simulink model "linear2DOF"  (R2025b)
settings: Solver=FixedStepAuto  StartTime=0.0  StopTime=1000  FixedStep=0.001  RelTol=1e-3
InitFcn:
  | % 定义车辆参数
  | m = 1370 + 89.9 + 65.2 + 22*4;       % 车辆质量 (kg)
  | Vx = 120/3.6;        % 纵向速度 (m/s)
  | Cf = -4.487763550086564e+04 * 2;    % 前轴总侧偏刚度 (N/rad)
  | Cr = Cf;   % 后轴总侧偏刚度 (N/rad)
  | lf = 1.11;       % 质心到前轴距离 (m)
  | lr = 2.866-lf;       % 质心到后轴距离 (m)
  | Iz = 2315.3 + 0.08 + 0.08 + 0.8*4;      % 绕z轴转动惯量 (kg·m²)
undefined symbols (not defined in the file): speed_from_matlab
libraries: Solver_SF x1
settings Model: Creator=23649  LastModifiedBy=23649

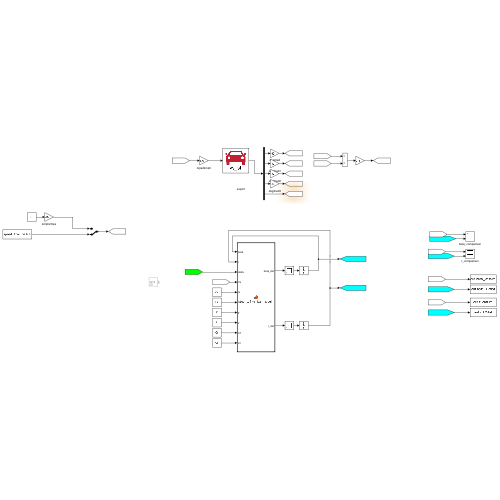
[thumbnail: Simulink's stored preview of the top-level diagram]
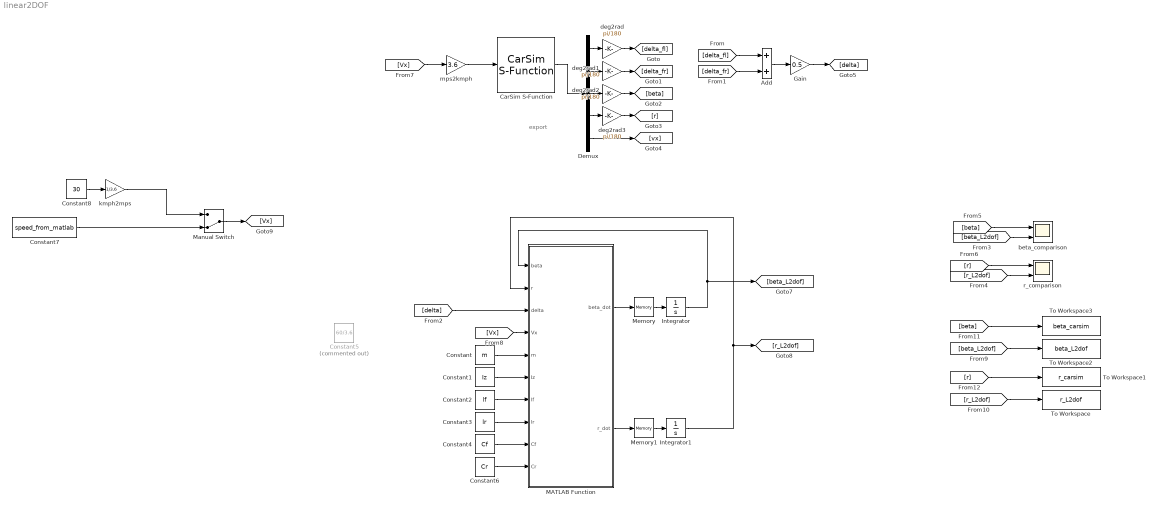
== system linear2DOF ==
  note: export
  Add : Sum
  CarSim S-Function : Solver_SF/CarSim S-Function  Priority=1  SIMFILE=simfile.sim  Run_RTs=off  vs_state_ind=Run  StopMode_ind=Vehicle Model
  Constant : Constant  Value=m
  Constant1 : Constant  Value=Iz
  Constant2 : Constant  Value=lf
  Constant3 : Constant  Value=lr
  Constant4 : Constant  Value=Cf
  Constant5 : Constant  Commented=on  Value=60/3.6
  Constant6 : Constant  Value=Cr
  Constant7 : Constant  Value=speed_from_matlab
  Constant8 : Constant  Value=30
  Demux : Demux  Outputs=5
  Gain : Gain  Gain=0.5
  Integrator : Integrator
  Integrator1 : Integrator
  MATLAB Function : MATLAB Function  TreatAsAtomicUnit=on
  Manual Switch : ManualSwitch  CurrentSetting=0
  Memory : Memory
  Memory1 : Memory
  To Workspace : ToWorkspace  VariableName=r_L2dof  SampleTime=-1
  To Workspace1 : ToWorkspace  VariableName=r_carsim  SampleTime=-1
  To Workspace2 : ToWorkspace  VariableName=beta_L2dof  SampleTime=-1
  To Workspace3 : ToWorkspace  VariableName=beta_carsim  SampleTime=-1
  beta_comparison : Scope  NumInputPorts=2
      settings: ActiveDisplayYMinimum=-1  ActiveDisplayYMaximum=1
  deg2rad{,1..3} (4 alike) : Gain  Gain=pi/180
  kmph2mps : Gain  Gain=1/3.6
  mps2kmph : Gain  Gain=3.6
  r_comparison : Scope  NumInputPorts=2
      settings: ActiveDisplayYMinimum=-0.23111502983023319  ActiveDisplayYMaximum=0.23036236303418919
  wires:
  CarSim S-Function/1 -> Demux/1
  Demux/5 -> [vx]
  Demux/4 -> deg2rad3/1
  Demux/3 -> deg2rad2/1
  Demux/2 -> deg2rad1/1
  Demux/1 -> deg2rad/1
  deg2rad/1 -> [delta_fl]
  deg2rad1/1 -> [delta_fr]
  [delta_fl] -> Add/1
  Add/1 -> Gain/1
  [delta_fr] -> Add/2
  Gain/1 -> [delta]
  [delta] -> MATLAB Function/3(delta)
  MATLAB Function/1(beta_dot) -> Memory/1
  MATLAB Function/2(r_dot) -> Memory1/1
  Memory/1 -> Integrator/1
  Memory1/1 -> Integrator1/1
  Integrator/1 -> MATLAB Function/1(beta), [beta_L2dof]
  Integrator1/1 -> [r_L2dof], MATLAB Function/2(r)
  [Vx] -> MATLAB Function/4(Vx)
  Constant6/1 -> MATLAB Function/10(Cr)
  Constant4/1 -> MATLAB Function/9(Cf)
  Constant3/1 -> MATLAB Function/8(lr)
  Constant2/1 -> MATLAB Function/7(lf)
  Constant1/1 -> MATLAB Function/6(Iz)
  Constant/1 -> MATLAB Function/5(m)
  [r] -> r_comparison/1
  [r_L2dof] -> r_comparison/2
  deg2rad2/1 -> [beta]
  deg2rad3/1 -> [r]
  [beta] -> beta_comparison/1
  [beta_L2dof] -> beta_comparison/2
  [Vx] -> mps2kmph/1
  Constant8/1 -> kmph2mps/1
  mps2kmph/1 -> CarSim S-Function/1
  Manual Switch/1 -> [Vx]
  kmph2mps/1 -> Manual Switch/1
  Constant7/1 -> Manual Switch/2
  [r_L2dof] -> To Workspace/1
  [r] -> To Workspace1/1
  [beta] -> To Workspace3/1
  [beta_L2dof] -> To Workspace2/1

== matlab function linear2DOF/MATLAB Function ==
  data: beta input; r input; delta input; Vx input; beta_dot output; r_dot output; m input; Iz input; lf input; lr input; Cf input; Cr input
function [beta_dot, r_dot] = two_dof_vehicle_model(beta, r, delta, Vx, m, Iz, lf, lr, Cf, Cr)
    % 线性二自由度车辆动力学模型
    % 输入：
    %   β: 质心侧偏角 (rad)
    %   r: 横摆角速度 (rad/s)
    %   delta：前轮转角 (rad)
    %   Vx: 纵向速度 (m/s)
    %   整车params - 参数结构体，包含：
    %       m: 车辆质量 (kg)
    %       Iz: 绕z轴转动惯量 (kg·m²)
    %       lf: 质心到前轴距离 (m)
    %       lr: 质心到后轴距离 (m)
    %       Cf: 前轴总侧偏刚度 (N/rad)
    %       Cr: 后轴总侧偏刚度 (N/rad)
    % 输出：
    %   beta_dot, r_dot - 状态导数 [dβ/dt; dr/dt]
  
    
    % 计算状态导数
    beta_dot = (Cf + Cr)/(m * Vx) * beta + ...
               ((Cf * lf - Cr * lr)/(m * Vx^2) - 1) * r - ...
               (Cf/(m * Vx)) * delta;
    
    r_dot = (lf * Cf - lr * Cr)/Iz * beta + ...
            (lf^2 * Cf + lr^2 * Cr)/(Iz * Vx) * r - ...
            (lf * Cf)/Iz * delta;
    
end
